simulink model "modelTest"  (R2021b)
settings: Solver=VariableStepAuto  StartTime=0.0  StopTime=100.0  RelTol=1e-3
values from neighbouring files (symbols this model uses):
  deltaE_trim = -0.0836    [ConstFile.mat]    (also in script.m = ConstStruct.deltaE_trim)
  deltaT_trim = 0.499    [ConstFile.mat]    (also in script.m = ConstStruct.deltaT_trim)
settings Model: Creator=jacob  LastModifiedBy=jacob

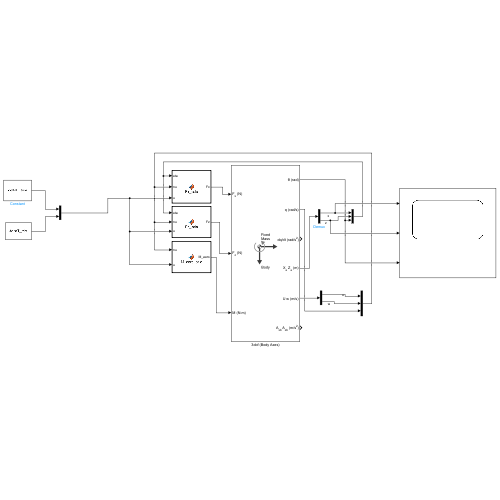
[thumbnail: Simulink's stored preview of the top-level diagram]
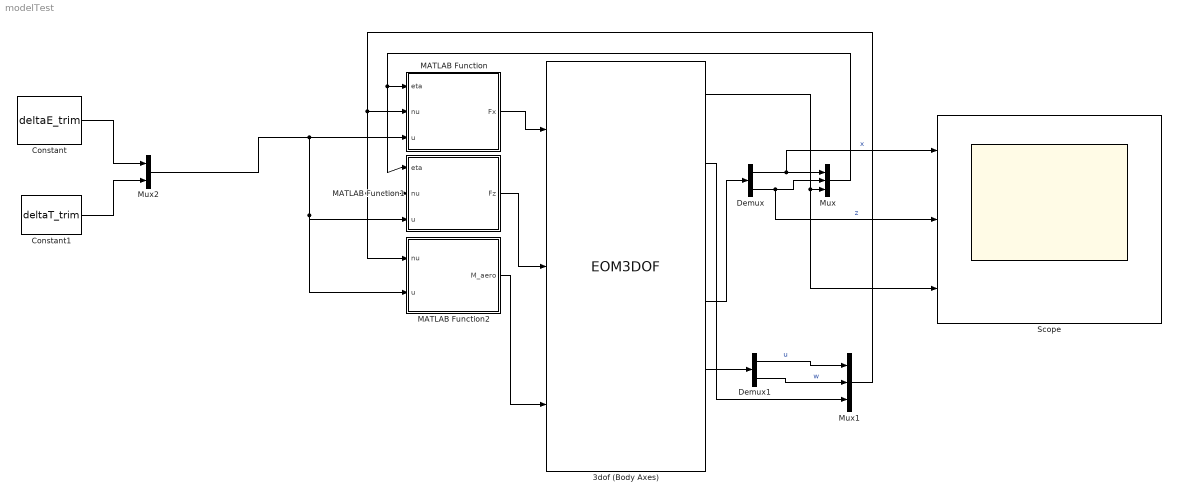
== system modelTest ==
  3dof (Body Axes) : EOM3DOF  v_ini=Va_trim  theta_ini=theta_trim  mass=m  Iyy=Jy
  Constant : Constant  Value=deltaE_trim
  Constant1 : Constant  Value=deltaT_trim
  Demux : Demux  Outputs=2
  Demux1 : Demux  Outputs=2
  MATLAB Function : MATLAB Function  TreatAsAtomicUnit=on
  MATLAB Function1 : MATLAB Function  TreatAsAtomicUnit=on
  MATLAB Function2 : MATLAB Function  TreatAsAtomicUnit=on
  Mux : Mux  Inputs=3
  Mux1 : Mux  Inputs=3
  Mux2 : Mux  Inputs=2
  Scope : Scope  NumInputPorts=3
  wires:
  MATLAB Function/1(Fx) -> 3dof (Body Axes)/1
  MATLAB Function1/1(Fz) -> 3dof (Body Axes)/2
  MATLAB Function2/1(M_aero) -> 3dof (Body Axes)/3
  3dof (Body Axes)/4 -> Demux/1
  Demux/1 -> Scope/1, Mux/1  "x"
  Demux/2 -> Scope/2, Mux/2  "z"
  3dof (Body Axes)/1 -> Scope/3, Mux/3
  Mux/1 -> MATLAB Function1/1(eta), MATLAB Function/1(eta)
  3dof (Body Axes)/5 -> Demux1/1
  Demux1/1 -> Mux1/1  "u"
  Demux1/2 -> Mux1/2  "w"
  3dof (Body Axes)/2 -> Mux1/3
  Mux1/1 -> MATLAB Function2/1(nu), MATLAB Function1/2(nu), MATLAB Function/2(nu)
  Constant/1 -> Mux2/1
  Constant1/1 -> Mux2/2
  Mux2/1 -> MATLAB Function2/2(u), MATLAB Function1/3(u), MATLAB Function/3(u)

== matlab function modelTest/MATLAB Function ==
  data: eta input; nu input; u input; Fx output
function Fx = Fx_calc(eta,nu,u)
h = 0.0001; %timestep
iterations = 1000000;

% ship parameters
m = 25;          % mass (kg)
Jy = 2.135;         % pitch moment of inertia (kg m^3)
xg = 0;              % CG x-ccordinate (m)

% Aero parameters
rho = 1.2682; %air density
alpha_0 = 0.4712; %rad
M = 50; %blending factor in aero coefficient calculation taken from beard&McLain appendix E

CL0 = 0.23; % Coefficient of lift at 0 pitch taken from beard&McLain appendix E
CL_alpha = -0.98;%5.61; %Derivative of CL wrt. alpha taken from beard&McLain appendix E
CL_q = 0;%7.95; %Derivative of CL wrt. q taken from beard&McLain appendix E
CL_deltaE = -0.36;%0.13; %Derivative of CL wrt. deltaE taken from beard&McLain appendix E

CD0 = 0.043; % Coefficient of drag
CD_alpha = 0.03; %Derivative of CD wrt. alpha taken from beard&McLain appendix E
CD_q = 0; %Derivative of CD wrt. q taken from beard&McLain appendix E
CD_deltaE = 0;%0.0135; %Derivative of CD wrt. deltaE taken from beard&McLain appendix E
CD_p = 0;

CM0 = 0.0135; % Aero moment coefficient
CM_alpha = -2.74; %0.38 %Derivative of CM wrt. alpha taken from beard&McLain appendix E
CM_q = -38.21; %Derivative of CM wrt. q taken from beard&McLain appendix E
CM_deltaE = -0.99; %Derivative of CM wrt. deltaE taken from beard&McLain appendix E

S = 0.55;  %Wing area taken from beard&McLain appendix E
c = 0.18994;  %moment arm for wing taken from beard&McLain appendix E
b = 2.8956;%wingspan taken from beard&McLain appendix E
e = 0.9;
g = 9.81;

S_prop = 0.2027;%taken from beard&McLain appendix E
C_prop = 1; %just tuning here?
k_motor = 80; %taken from beard&McLain appendix E

deltaE_trim = -0.0836;
deltaT_trim = 0.4990;
u_trim = 38.1551; %using Va = 40 and gamma = 0 in trim
w_trim = 1.8510;
theta_trim = 0.0485;
Va_trim = 38.2;
gamma_trim = 0;
alpha_trim = 0.0485;
q_trim = 0;

Va = sqrt(nu(1)*nu(1)+ nu(2)*nu(2));
theta = eta(3);
q = nu(3);
alpha = atan2(nu(2),nu(1));%angle of attack

% CONTROL


deltaT = u(1);
deltaE = u(2);

R_inertial_to_body = [cos(theta), -sin(theta);
    sin(theta), cos(theta)]; %Rotation matrix from body to inertial



R_stab_to_body = [cos(alpha),-sin(alpha);
    sin(alpha), cos(alpha)]; %rotation from stability to body

%Compute gravity
FG = R_inertial_to_body*[0; m*9.81];

Fx_G = 0;%FG(1);
Fz_G = 0;%FG(2);

%Compute propeller thrust
Fx_thrust=0.5*rho*S_prop*C_prop*((k_motor*deltaT)*(k_motor*deltaT)-Va*Va);


[CL_ofAlpha, CD_ofAlpha] = computeAeroCoeffs(alpha, alpha_0, M, S, b, e, CL0, CD_p);


CL = CL_ofAlpha + CL_q * 0.5*c*q/Va + CL_deltaE*deltaE;
CD = CD_ofAlpha + CD_q * 0.5*c*q/Va + CD_deltaE*deltaE;

F_lift = 0.5*rho*Va*Va*S*CL;
F_drag = 0.5*rho*Va*Va*S*CD;

CM = CM0 + CM_alpha * alpha + CM_deltaE*deltaE + CM_q*0.5*c*q/Va;
M_aero = 0.5*rho*Va*Va*S*c*CM;


F_aero = R_stab_to_body * [-F_drag;-F_lift]; %Transform to body frame

Fx_aero = F_aero(1);
Fz_aero = F_aero(2);

fx = Fx_G - Fx_aero + Fx_thrust;
fz = -Fz_G - Fz_aero;


CRB = nu(3)*[0, -1, 0;
    1, 0, 0;
    0, 0, 0];

F = [fx/m; fz/m; M_aero/Jy];


Fx = fx;

end

== matlab function modelTest/MATLAB Function2 ==
  data: nu input; u input; M_aero output
function M_aero = M_aero_calc(nu,u)

% Aero parameters
rho = 1.2682; %air density
CM0 = 0.0135; % Aero moment coefficient
CM_alpha = -2.74; %0.38 %Derivative of CM wrt. alpha taken from beard&McLain appendix E
CM_q = -38.21; %Derivative of CM wrt. q taken from beard&McLain appendix E
CM_deltaE = -0.99; %Derivative of CM wrt. deltaE taken from beard&McLain appendix E
S = 0.55;  %Wing area taken from beard&McLain appendix E
c = 0.18994;  %moment arm for wing taken from beard&McLain appendix E

%-------------%
Va = sqrt(nu(1)*nu(1)+ nu(2)*nu(2));
q = nu(3);
alpha = atan2(nu(2),nu(1));%angle of attack

% CONTROL

deltaE = u(2);

CM = CM0 + CM_alpha * alpha + CM_deltaE*deltaE + CM_q*0.5*c*q/Va;
M_aero = 0.5*rho*Va*Va*S*c*CM;


end

== matlab function modelTest/MATLAB Function1 ==
  data: eta input; nu input; u input; Fz output
function Fz = Fz_calc(eta,nu,u)
h = 0.0001; %timestep
iterations = 1000000;

% ship parameters
m = 25;          % mass (kg)
Jy = 2.135;         % pitch moment of inertia (kg m^3)
xg = 0;              % CG x-ccordinate (m)

% Aero parameters
rho = 1.2682; %air density
alpha_0 = 0.4712; %rad
M = 50; %blending factor in aero coefficient calculation taken from beard&McLain appendix E

CL0 = 0.23; % Coefficient of lift at 0 pitch taken from beard&McLain appendix E
CL_alpha = -0.98;%5.61; %Derivative of CL wrt. alpha taken from beard&McLain appendix E
CL_q = 0;%7.95; %Derivative of CL wrt. q taken from beard&McLain appendix E
CL_deltaE = -0.36;%0.13; %Derivative of CL wrt. deltaE taken from beard&McLain appendix E

CD0 = 0.043; % Coefficient of drag
CD_alpha = 0.03; %Derivative of CD wrt. alpha taken from beard&McLain appendix E
CD_q = 0; %Derivative of CD wrt. q taken from beard&McLain appendix E
CD_deltaE = 0;%0.0135; %Derivative of CD wrt. deltaE taken from beard&McLain appendix E
CD_p = 0;

CM0 = 0.0135; % Aero moment coefficient
CM_alpha = -2.74; %0.38 %Derivative of CM wrt. alpha taken from beard&McLain appendix E
CM_q = -38.21; %Derivative of CM wrt. q taken from beard&McLain appendix E
CM_deltaE = -0.99; %Derivative of CM wrt. deltaE taken from beard&McLain appendix E

S = 0.55;  %Wing area taken from beard&McLain appendix E
c = 0.18994;  %moment arm for wing taken from beard&McLain appendix E
b = 2.8956;%wingspan taken from beard&McLain appendix E
e = 0.9;
g = 9.81;

S_prop = 0.2027;%taken from beard&McLain appendix E
C_prop = 1; %just tuning here?
k_motor = 80; %taken from beard&McLain appendix E

deltaE_trim = -0.0836;
deltaT_trim = 0.4990;
u_trim = 38.1551; %using Va = 40 and gamma = 0 in trim
w_trim = 1.8510;
theta_trim = 0.0485;
Va_trim = 38.2;
gamma_trim = 0;
alpha_trim = 0.0485;
q_trim = 0;

Va = sqrt(nu(1)*nu(1)+ nu(2)*nu(2));
theta = eta(3);
q = nu(3);
alpha = atan2(nu(2),nu(1));%angle of attack

% CONTROL


deltaT = u(1);
deltaE = u(2);

R_inertial_to_body = [cos(theta), -sin(theta);
    sin(theta), cos(theta)]; %Rotation matrix from body to inertial



R_stab_to_body = [cos(alpha),-sin(alpha);
    sin(alpha), cos(alpha)]; %rotation from stability to body

%Compute gravity
FG = R_inertial_to_body*[0; m*9.81];

Fx_G = 0;%FG(1);
Fz_G = 0;%FG(2);

%Compute propeller thrust
Fx_thrust=0.5*rho*S_prop*C_prop*((k_motor*deltaT)*(k_motor*deltaT)-Va*Va);


[CL_ofAlpha, CD_ofAlpha] = computeAeroCoeffs(alpha, alpha_0, M, S, b, e, CL0, CD_p);


CL = CL_ofAlpha + CL_q * 0.5*c*q/Va + CL_deltaE*deltaE;
CD = CD_ofAlpha + CD_q * 0.5*c*q/Va + CD_deltaE*deltaE;

F_lift = 0.5*rho*Va*Va*S*CL;
F_drag = 0.5*rho*Va*Va*S*CD;

CM = CM0 + CM_alpha * alpha + CM_deltaE*deltaE + CM_q*0.5*c*q/Va;
M_aero = 0.5*rho*Va*Va*S*c*CM;


F_aero = R_stab_to_body * [-F_drag;-F_lift]; %Transform to body frame

Fx_aero = F_aero(1);
Fz_aero = F_aero(2);

fx = Fx_G - Fx_aero + Fx_thrust;
fz = -Fz_G - Fz_aero;


CRB = nu(3)*[0, -1, 0;
    1, 0, 0;
    0, 0, 0];

F = [fx/m; fz/m; M_aero/Jy];


Fz = fz;

end
